simulink model "carsim_brake_cosim"  (R2024b)
settings: Solver=ode45  StartTime=0.0  StopTime=6  FixedStep=0.002  RelTol=1e-3
undefined symbols (not defined in the file or in its folder): case_mu
libraries: Solver_SF x1
settings Model: Creator=MrZang  LastModifiedBy=MrZang
settings DataIOCC: SignalLogging=off

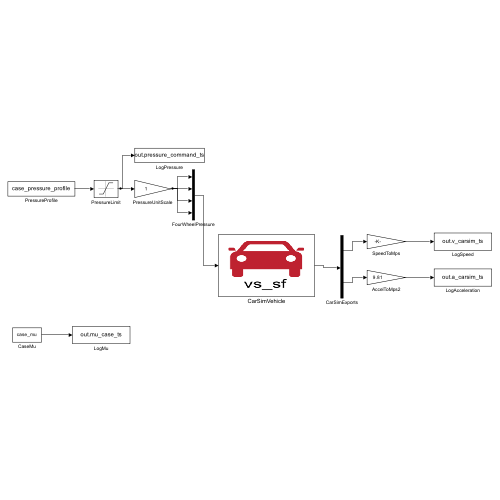
[thumbnail: Simulink's stored preview of the top-level diagram]
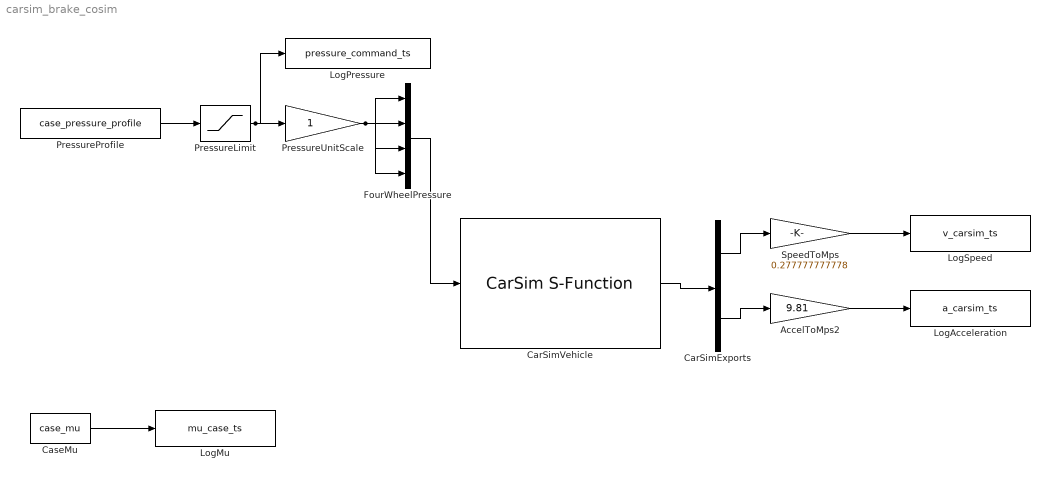
== system carsim_brake_cosim ==
  AccelToMps2 : Gain  Gain=9.81
  CarSimExports : Demux  Outputs=2
  CarSimVehicle : Solver_SF/CarSim S-Function  Priority=1  SIMFILE=F:\Carsim\UserData\simfile.sim
  CaseMu : Constant  Value=case_mu
  FourWheelPressure : Mux
  LogAcceleration : ToWorkspace  VariableName=a_carsim_ts  SaveFormat=Timeseries  SampleTime=-1
  LogMu : ToWorkspace  VariableName=mu_case_ts  SaveFormat=Timeseries  SampleTime=-1
  LogPressure : ToWorkspace  VariableName=pressure_command_ts  SaveFormat=Timeseries  SampleTime=-1
  LogSpeed : ToWorkspace  VariableName=v_carsim_ts  SaveFormat=Timeseries  SampleTime=-1
  PressureLimit : Saturate  UpperLimit=10  LowerLimit=0
  PressureProfile : FromWorkspace  VariableName=case_pressure_profile  OutputAfterFinalValue=Holding final value
  PressureUnitScale : Gain
  SpeedToMps : Gain  Gain=0.277777777778
  wires:
  PressureProfile/1 -> PressureLimit/1
  PressureLimit/1 -> PressureUnitScale/1, LogPressure/1
  PressureUnitScale/1 -> FourWheelPressure/1, FourWheelPressure/2, FourWheelPressure/3, FourWheelPressure/4
  FourWheelPressure/1 -> CarSimVehicle/1
  CarSimVehicle/1 -> CarSimExports/1
  CarSimExports/1 -> SpeedToMps/1
  CarSimExports/2 -> AccelToMps2/1
  SpeedToMps/1 -> LogSpeed/1
  AccelToMps2/1 -> LogAcceleration/1
  CaseMu/1 -> LogMu/1
